simulink model "w3_prob1_214869"  (R2020a)
settings: Solver=VariableStepAuto  StartTime=0.0  StopTime=10.0  RelTol=1e-3
settings Model: Creator=sonal  LastModifiedBy=sonal

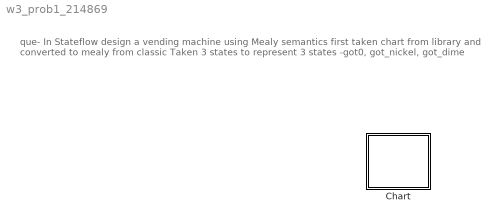
== system w3_prob1_214869 ==
  note: que- In Stateflow design a vending machine using Mealy semantics
      | first taken chart from library and converted to mealy from classic
      | Taken 3 states to represent 3 states -got0, got_nickel, got_dime
  Chart : Stateflow chart  TreatAsAtomicUnit=on

== stateflow chart w3_prob1_214869/Chart ==
  settings: stateMachineType=MEALY_MACHINE
  state ?
  state ?
  state ?
  (default) -> ?
